simulink model "Control_Loop_illustration"  (R2021a)
settings: Solver=VariableStepAuto  StartTime=0.0  StopTime=10.0  RelTol=1e-3
settings Model: Creator=ornul  LastModifiedBy=ornul

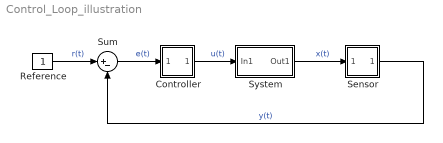
== system Control_Loop_illustration ==
  Controller : Subsystem
  Reference : Constant
  Sensor : Subsystem
  Sum : Sum  Inputs=|+-
  System : Subsystem
  wires:
  Reference/1 -> Sum/1  "r(t)"
  Sum/1 -> Controller/1(In1)  "e(t)"
  Controller/1(Out1) -> System/1(In1)  "u(t)"
  System/1(Out1) -> Sensor/1(In1)  "x(t)"
  Sensor/1(Out1) -> Sum/2  "y(t)"

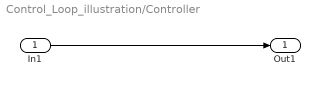
== system Control_Loop_illustration/Controller ==
  In1 : Inport
  Out1 : Outport
  wires:
  In1/1 -> Out1/1

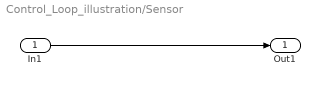
== system Control_Loop_illustration/Sensor ==
  In1 : Inport
  Out1 : Outport
  wires:
  In1/1 -> Out1/1

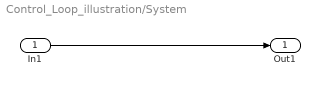
== system Control_Loop_illustration/System ==
  In1 : Inport
  Out1 : Outport
  wires:
  In1/1 -> Out1/1
